simulink model "signal"  (R2021b)
settings: Solver=FixedStepAuto  StartTime=0.0  StopTime=1  FixedStep=0.01  RelTol=1e-3
libraries: mcbhostblockslib x3
settings Model: Creator=anton  LastModifiedBy=anton

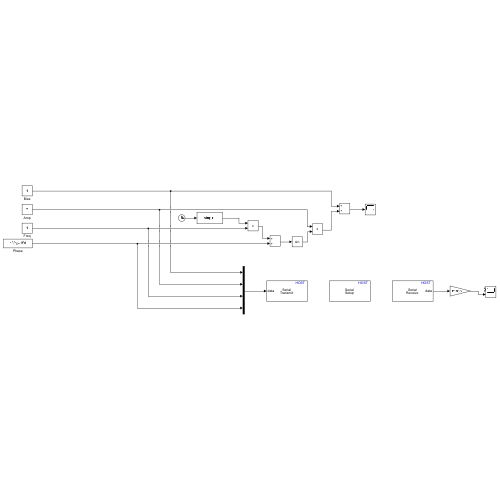
[thumbnail: Simulink's stored preview of the top-level diagram]
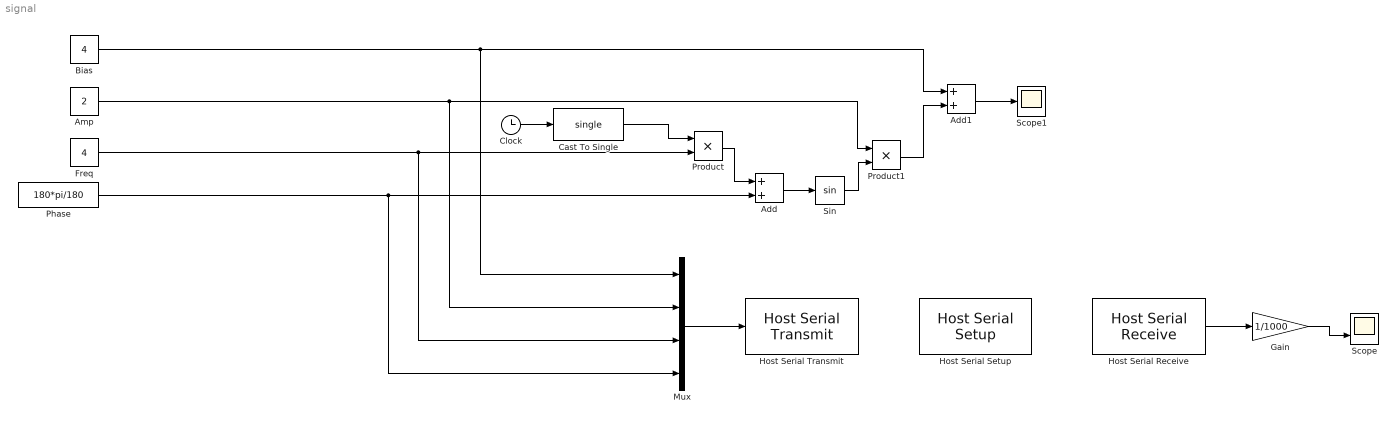
== system signal ==
  Add : Sum
  Add1 : Sum
  Amp : Constant  Value=2  OutDataTypeStr=uint8
  Bias : Constant  Value=4  OutDataTypeStr=uint8
  Cast To Single : DataTypeConversion  OutDataTypeStr=single
  Clock : Clock
  Freq : Constant  Value=4  OutDataTypeStr=uint8
  Gain : Gain  Gain=1/1000
  Host Serial Receive : mcbhostblockslib/Host Serial Receive  serialCon=Serial 1  dataHead='SSSS'  dataTail='EEEE'  dataType=int32  dataDim=[1 1]  initValue=0  errOption=Output the last received value  errValue=0  sampleTime=-1  outputStatus=off  blockingMode=on
      settings: SourceProductBaseCode=MT
  Host Serial Setup : mcbhostblockslib/Host Serial Setup  Priority=-99  comPortSer1='COM11'  baudRateA=115200  charLenA=8  stopBitA=1  parityA=none  timeoutA=1  ByteOrderA=LittleEndian  comPortSer2='Please_select_a_port'  baudRateB=115200  charLenB=8  stopBitB=1  parityB=none  timeoutB=1.0  ByteOrderB=LittleEndian  comPortSer3='Please_select_a_port'  baudRateC=115200  charLenC=8  stopBitC=1  parityC=none  timeoutC=1.0  ByteOrderC=LittleEndian  comPortSer4='Please_select_a_port'  baudRateD=115200  charLenD=8  stopBitD=1  parityD=none  timeoutD=1.0  ByteOrderD=LittleEndian
      settings: SourceProductBaseCode=MT
  Host Serial Transmit : mcbhostblockslib/Host Serial Transmit  serialCon=Serial 1  header='S'  tail='E'  enableBlockingMode=off
      settings: SourceProductBaseCode=MT
  Mux : Mux
  Phase : Constant  Value=180*pi/180  OutDataTypeStr=uint8
  Product : Product
  Product1 : Product
  Scope : Scope  NumInputPorts=2
  Scope1 : Scope
  Sin : Trigonometry
  wires:
  Clock/1 -> Cast To Single/1
  Product/1 -> Add/1
  Add/1 -> Sin/1
  Sin/1 -> Product1/2
  Product1/1 -> Add1/2
  Add1/1 -> Scope1/1
  Mux/1 -> Host Serial Transmit/1
  Cast To Single/1 -> Product/1
  Phase/1 -> Mux/4, Add/2
  Freq/1 -> Product/2, Mux/3
  Amp/1 -> Product1/1, Mux/2
  Bias/1 -> Add1/1, Mux/1
  Host Serial Receive/1 -> Gain/1
  Gain/1 -> Scope/2
